simulink model "PV_model_Param"  (Simulink 7.9)
settings: Solver=VariableStepDiscrete  StartTime=0.0  StopTime=0.1  MaxStep=20e-6  RelTol=1e-3
undefined symbols (not defined in the file): Iph, Isat, Rp, Rs, Voc, VT
libraries: simulink x1
settings Model: Creator=Gilbert  LastModifiedBy=by2815
settings DebuggingCC: AlgebraicLoopMsg=none
settings GRTTargetCC: CombineOutputUpdateFcns=off  GRTInterface=on

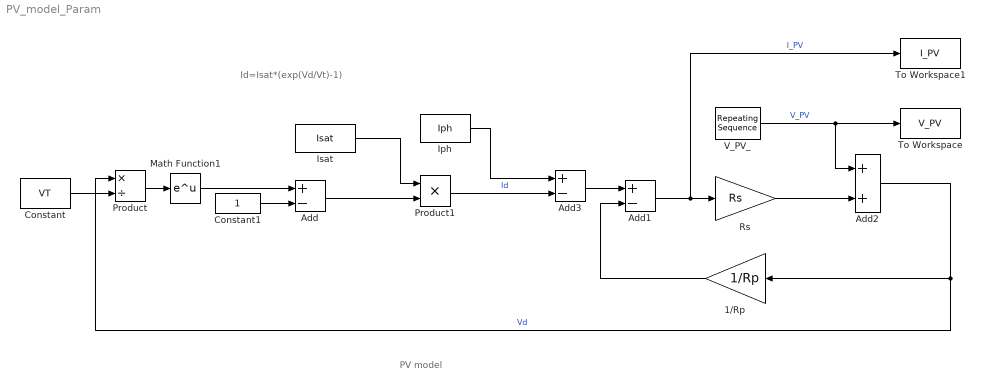
== system PV_model_Param ==
  note: PV model
  note: Id=Isat*(exp(Vd/Vt)-1)
  1/Rp : Gain  Gain=1/Rp
  Add : Sum  Inputs=+-
  Add1 : Sum  Inputs=+-
  Add2 : Sum
  Add3 : Sum  Inputs=+-
  Constant : Constant  Value=VT
  Constant1 : Constant
  Iph : Constant  Value=Iph
  Isat : Constant  Value=Isat
  Math Function1 : Math  SaturateOnIntegerOverflow=on
  Product : Product  Inputs=*/  RndMeth=Zero
  Product1 : Product  Inputs=**  RndMeth=Zero
  Rs : Gain  Gain=Rs
  To Workspace : ToWorkspace  VariableName=V_PV  SampleTime=-1
  To Workspace1 : ToWorkspace  VariableName=I_PV  SampleTime=-1
  V_PV_ : simulink/Sources/Repeating Sequence  rep_seq_t=[0 0.1 0.2]  rep_seq_y=[0 Voc 0]
  wires:
  Constant/1 -> Product/2
  Constant1/1 -> Add/2
  Add/1 -> Product1/2
  Isat/1 -> Product1/1
  1/Rp/1 -> Add1/2
  Add1/1 -> Rs/1, To Workspace1/1  "I_PV"
  Rs/1 -> Add2/2
  Add2/1 -> 1/Rp/1, Product/1  "Vd"
  Add3/1 -> Add1/1
  Product1/1 -> Add3/2  "Id"
  Iph/1 -> Add3/1
  V_PV_/1 -> Add2/1, To Workspace/1  "V_PV"
  Product/1 -> Math Function1/1
  Math Function1/1 -> Add/1
